simulink model "chap02_03_36_mdl"  (R2013b)
settings: Solver=ode4  StartTime=0.0  StopTime=inf  FixedStep=0.1  RelTol=1e-3
settings Model: Creator=Administrator  LastModifiedBy=sunzx.fnst

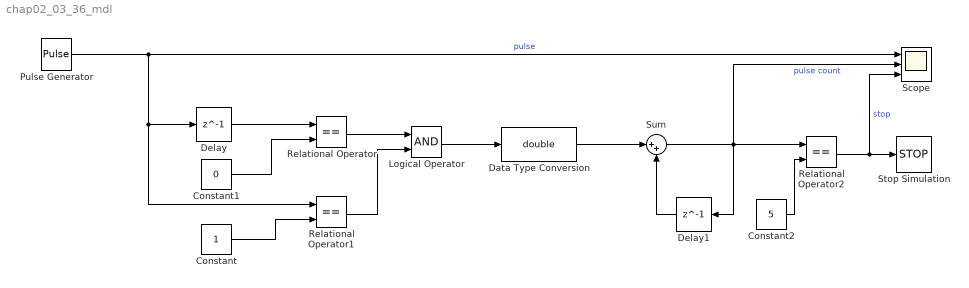
== system chap02_03_36_mdl ==
  Constant : Constant
  Constant1 : Constant  Value=0
  Constant2 : Constant  Value=5
  Data Type Conversion : DataTypeConversion  OutDataTypeStr=double
  Delay : Delay  DelayLength=1  InitialCondition=0
  Delay1 : Delay  DelayLength=1  InitialCondition=0
  Logical Operator : Logic  AllPortsSameDT=off  OutDataTypeStr=boolean
  Pulse Generator : DiscretePulseGenerator  PulseType=Time based  PulseWidth=50  PhaseDelay=0.2
  Relational Operator : RelationalOperator  Operator===  OutDataTypeStr=boolean
  Relational Operator1 : RelationalOperator  Operator===  OutDataTypeStr=boolean
  Relational Operator2 : RelationalOperator  Operator===  OutDataTypeStr=boolean
  Scope : Scope  NumInputPorts=3
      settings: YMin=-5~-5~-5  YMax=5~5~5
  Stop Simulation : Stop
  Sum : Sum  Inputs=|++
  wires:
  Pulse Generator/1 -> Relational Operator1/1, Delay/1, Scope/1  "pulse"
  Constant/1 -> Relational Operator1/2
  Delay/1 -> Relational Operator/1
  Constant1/1 -> Relational Operator/2
  Relational Operator/1 -> Logical Operator/1
  Relational Operator1/1 -> Logical Operator/2
  Logical Operator/1 -> Data Type Conversion/1
  Delay1/1 -> Sum/2
  Sum/1 -> Relational Operator2/1, Delay1/1, Scope/2  "pulse count"
  Relational Operator2/1 -> Scope/3, Stop Simulation/1  "stop"
  Constant2/1 -> Relational Operator2/2
  Data Type Conversion/1 -> Sum/1
